simulink model "mpc_test"  (R2021b)
settings: Solver=VariableStepAuto  StartTime=0.0  StopTime=14  RelTol=1e-3
undefined symbols (not defined in the file or in its folder): carb1, carb2, carb3, carb4, carb5, DIM, KLa1, KLa2, KLa3, KLa4, LAYER, MODELTYPE, PAR1, PAR2, PAR3, PAR4, PAR5, Qin0, SETTLERINIT, SETTLERPAR, SNO2ref, SO5ref, SOSAT1, SOSAT2, SOSAT3, SOSAT4, SOSAT5, SparrowMPC_Control, T, VOL1, VOL2, VOL3, VOL4, VOL5, XINIT1, XINIT2, XINIT3, XINIT4, XINIT5, XINITDELAY
settings Model: SimulationMode=accelerator  Creator=匡  LastModifiedBy=匡
settings SolverCC: AlgebraicLoopSolver=TrustRegion
settings DataIOCC: ReturnWorkspaceOutputs=off  OutputOption=SpecifiedOutputTimes  OutputTimes=[0:1/96:14]
settings OptimizationCC: EfficientMapNaN2IntZero=off
settings DebuggingCC: InheritedTsInSrcMsg=none  UnknownTsInhSupMsg=none  SFMachineParentedDataDiag=warning  ArithmeticOperatorsInVariantConditions=warning
settings HardwareCC: TargetBitPerPointer=64  TargetBitPerSizeT=64  TargetBitPerPtrDiffT=64  TargetLongLongMode=on  TargetIntDivRoundTo=Zero  TargetEndianess=LittleEndian  TargetWordSize=64  TargetHWDeviceType=MATLAB Host  ProdEqTarget=off
settings SFSimCC: SimUseLocalCustomCode=off  CustomCodeUndefinedFunction=UseInterfaceOnly
settings RTWCC: RTWUseLocalCustomCode=off
settings CodeAppCC: MaxIdLength=128
settings GRTTargetCC: TargetLangStandard=C89/C90 (ANSI)  CombineOutputUpdateFcns=off  GRTInterface=on

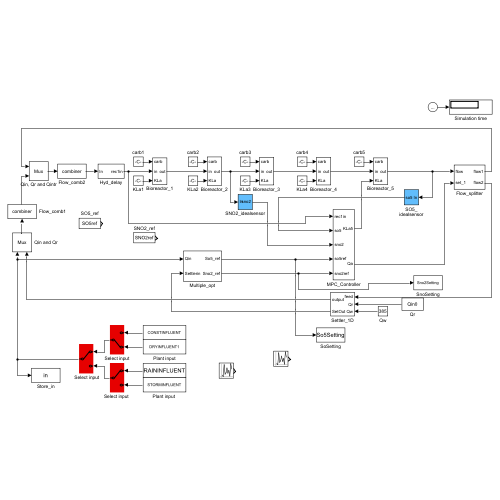
[thumbnail: Simulink's stored preview of the top-level diagram]
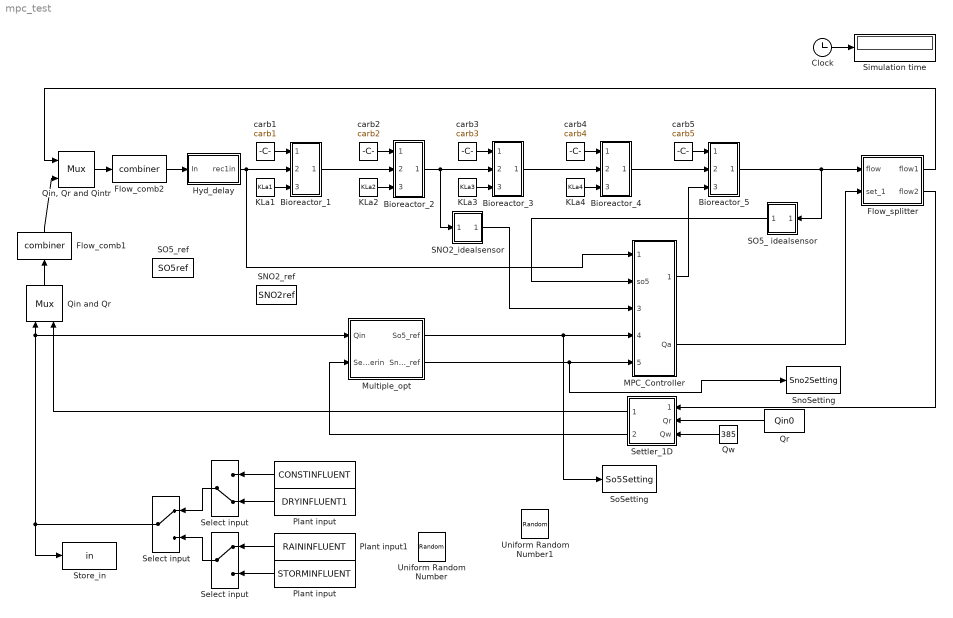
== system mpc_test ==
  " " : FromWorkspace  VariableName=CONSTINFLUENT  OutDataTypeStr=double  SampleTime=-1  ZeroCross=off  OutputAfterFinalValue=Holding final value
  " Select input" : ManualSwitch
  Bioreactor_1 : Subsystem
  Bioreactor_2 : Subsystem
  Bioreactor_3 : Subsystem
  Bioreactor_4 : Subsystem
  Bioreactor_5 : Subsystem
  Clock : Clock
  Flow_comb1 : S-Function  FunctionName=combiner  SFunctionDeploymentMode=off  EnableBusSupport=off
  Flow_comb2 : S-Function  FunctionName=combiner  SFunctionDeploymentMode=off  EnableBusSupport=off
  Flow_splitter : Subsystem
  Hyd_delay : Subsystem
  KLa1 : Constant  Value=KLa1
  KLa2 : Constant  Value=KLa2
  KLa3 : Constant  Value=KLa3
  KLa4 : Constant  Value=KLa4
  MPC_Controller : Subsystem
  Multiple_opt : Subsystem
  Plant input : FromWorkspace  VariableName=DRYINFLUENT1  SampleTime=-1  ZeroCross=off  OutputAfterFinalValue=Holding final value
  "Plant input " : FromWorkspace  VariableName=STORMINFLUENT  SampleTime=-1  ZeroCross=off  OutputAfterFinalValue=Holding final value
  Plant input1 : FromWorkspace  VariableName=RAININFLUENT  SampleTime=-1  ZeroCross=off  OutputAfterFinalValue=Holding final value
  Qin and Qr : Mux  Inputs=2
  "Qin, Qr and Qintr" : Mux  Inputs=2
  Qr : Constant  Value=Qin0
  Qw : Constant  Value=385
  SNO2_idealsensor : Subsystem
  SNO2_ref : Constant  Value=SNO2ref
  SO5_ idealsensor : Subsystem
  SO5_ref : Constant  Value=SO5ref
  Select input : ManualSwitch  CurrentSetting=0
  "Select input " : ManualSwitch
  Settler_1D : Subsystem
  Simulation time : Display
  SnoSetting : ToWorkspace  VariableName=Sno2Setting  SampleTime=1/96
  SoSetting : ToWorkspace  VariableName=So5Setting  SampleTime=1/96
  Store_in : ToWorkspace  VariableName=in  SampleTime=-1
  Uniform Random Number : UniformRandomNumber  Minimum=0.5  Maximum=2.5  Seed=547314  SampleTime=1/12
  Uniform Random Number1 : UniformRandomNumber  Minimum=0.4  Maximum=2  Seed=48658  SampleTime=1/12
  carb1 : Constant  Value=carb1
  carb2 : Constant  Value=carb2
  carb3 : Constant  Value=carb3
  carb4 : Constant  Value=carb4
  carb5 : Constant  Value=carb5
  wires:
  Settler_1D/1(output) -> Qin and Qr/2
  KLa3/1 -> Bioreactor_3/3(KLa)
  Flow_comb1/1 -> "Qin, Qr and Qintr"/2
  "Qin, Qr and Qintr"/1 -> Flow_comb2/1
  carb3/1 -> Bioreactor_3/1(carb)
  Bioreactor_1/1(out) -> Bioreactor_2/2(in)
  carb2/1 -> Bioreactor_2/1(carb)
  Plant input1/1 -> "Select input "/1
  KLa1/1 -> Bioreactor_1/3(KLa)
  carb4/1 -> Bioreactor_4/1(carb)
  Qw/1 -> Settler_1D/3(Qw)
  Bioreactor_5/1(out) -> Flow_splitter/1(flow), SO5_ idealsensor/1(In)
  KLa2/1 -> Bioreactor_2/3(KLa)
  Qin and Qr/1 -> Flow_comb1/1
  carb1/1 -> Bioreactor_1/1(carb)
  KLa4/1 -> Bioreactor_4/3(KLa)
  " "/1 -> Select input/1
  Flow_splitter/2(flow2) -> Settler_1D/1(feed)
  Flow_comb2/1 -> Hyd_delay/1(In)
  Clock/1 -> Simulation time/1
  Bioreactor_4/1(out) -> Bioreactor_5/2(in)
  "Plant input "/1 -> "Select input "/2
  Qr/1 -> Settler_1D/2(Qr)
  "Select input "/1 -> " Select input"/2
  Bioreactor_2/1(out) -> Bioreactor_3/2(in), SNO2_idealsensor/1(In)
  Select input/1 -> " Select input"/1
  Bioreactor_3/1(out) -> Bioreactor_4/2(in)
  Plant input/1 -> Select input/2
  carb5/1 -> Bioreactor_5/1(carb)
  MPC_Controller/1(KLa5) -> Bioreactor_5/3(KLa)
  MPC_Controller/2(Qa) -> Flow_splitter/2(set_1)
  SNO2_idealsensor/1(sno2) -> MPC_Controller/3(sno2)
  Hyd_delay/1(rec1in) -> MPC_Controller/1(rec1in), Bioreactor_1/2(in)
  SO5_ idealsensor/1(so5) -> MPC_Controller/2(so5)
  " Select input"/1 -> Store_in/1, Multiple_opt/1(Qin), Qin and Qr/1
  Flow_splitter/1(flow1) -> "Qin, Qr and Qintr"/1
  Settler_1D/2(SetOut) -> Multiple_opt/2(Settlerin)
  Multiple_opt/1(So5_ref) -> SoSetting/1, MPC_Controller/4(so5ref)
  Multiple_opt/2(Sno2_ref) -> SnoSetting/1, MPC_Controller/5(sno2ref)

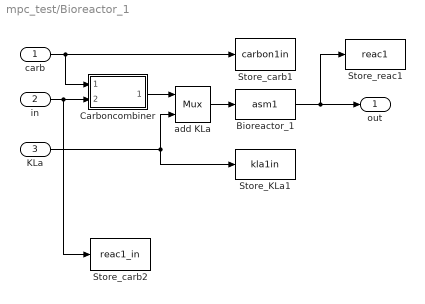
== system mpc_test/Bioreactor_1 ==
  carb : Inport
  in : Inport  Port=2
  KLa : Inport  Port=3
  Bioreactor_1 : S-Function  FunctionName=asm1  Parameters=XINIT1,PAR1,VOL1,SOSAT1  SFunctionDeploymentMode=off  EnableBusSupport=off
  Carboncombiner : Subsystem
  Store_KLa1 : ToWorkspace  VariableName=kla1in  SampleTime=-1
  Store_carb1 : ToWorkspace  VariableName=carbon1in  SampleTime=-1
  Store_carb2 : ToWorkspace  VariableName=reac1_in  SampleTime=-1
  Store_reac1 : ToWorkspace  VariableName=reac1  SampleTime=-1
  add KLa : Mux  Inputs=2
  out : Outport  VectorParamsAs1DForOutWhenUnconnected=off
  wires:
  add KLa/1 -> Bioreactor_1/1
  Bioreactor_1/1 -> out/1, Store_reac1/1
  Carboncombiner/1(Output) -> add KLa/1
  carb/1 -> Store_carb1/1, Carboncombiner/1(C_flow)
  in/1 -> Store_carb2/1, Carboncombiner/2(Input)
  KLa/1 -> add KLa/2, Store_KLa1/1

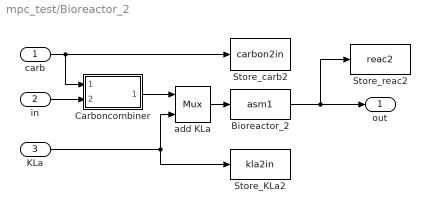
== system mpc_test/Bioreactor_2 ==
  carb : Inport
  in : Inport  Port=2
  KLa : Inport  Port=3
  Bioreactor_2 : S-Function  FunctionName=asm1  Parameters=XINIT2,PAR2,VOL2,SOSAT2  SFunctionDeploymentMode=off  EnableBusSupport=off
  Carboncombiner : Subsystem
  Store_KLa2 : ToWorkspace  VariableName=kla2in  SampleTime=-1
  Store_carb2 : ToWorkspace  VariableName=carbon2in  SampleTime=-1
  Store_reac2 : ToWorkspace  VariableName=reac2  SampleTime=-1
  add KLa : Mux  Inputs=2
  out : Outport  VectorParamsAs1DForOutWhenUnconnected=off
  wires:
  Bioreactor_2/1 -> out/1, Store_reac2/1
  add KLa/1 -> Bioreactor_2/1
  Carboncombiner/1(Output) -> add KLa/1
  carb/1 -> Carboncombiner/1(C_flow), Store_carb2/1
  in/1 -> Carboncombiner/2(Input)
  KLa/1 -> add KLa/2, Store_KLa2/1

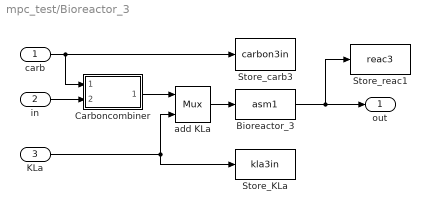
== system mpc_test/Bioreactor_3 ==
  carb : Inport
  in : Inport  Port=2
  KLa : Inport  Port=3
  Bioreactor_3 : S-Function  FunctionName=asm1  Parameters=XINIT3,PAR3,VOL3,SOSAT3  SFunctionDeploymentMode=off  EnableBusSupport=off
  Carboncombiner : Subsystem
  Store_KLa : ToWorkspace  VariableName=kla3in  SampleTime=-1
  Store_carb3 : ToWorkspace  VariableName=carbon3in  SampleTime=-1
  Store_reac1 : ToWorkspace  VariableName=reac3  SampleTime=-1
  add KLa : Mux  Inputs=2
  out : Outport  VectorParamsAs1DForOutWhenUnconnected=off
  wires:
  Bioreactor_3/1 -> out/1, Store_reac1/1
  add KLa/1 -> Bioreactor_3/1
  Carboncombiner/1(Output) -> add KLa/1
  carb/1 -> Carboncombiner/1(C_flow), Store_carb3/1
  in/1 -> Carboncombiner/2(Input)
  KLa/1 -> add KLa/2, Store_KLa/1

== system mpc_test/Bioreactor_4 ==
  carb : Inport
  in : Inport  Port=2
  KLa : Inport  Port=3
  Bioreactor_4 : S-Function  FunctionName=asm1  Parameters=XINIT4,PAR4,VOL4,SOSAT4  SFunctionDeploymentMode=off  EnableBusSupport=off
  Carboncombiner : Subsystem
  Store_KLa4 : ToWorkspace  VariableName=kla4in  SampleTime=-1
  Store_carb4 : ToWorkspace  VariableName=carbon4in  SampleTime=-1
  Store_reac4 : ToWorkspace  VariableName=reac4  SampleTime=-1
  add KLa : Mux  Inputs=2
  out : Outport  VectorParamsAs1DForOutWhenUnconnected=off
  wires:
  Bioreactor_4/1 -> out/1, Store_reac4/1
  add KLa/1 -> Bioreactor_4/1
  Carboncombiner/1(Output) -> add KLa/1
  carb/1 -> Carboncombiner/1(C_flow), Store_carb4/1
  in/1 -> Carboncombiner/2(Input)
  KLa/1 -> add KLa/2, Store_KLa4/1

== system mpc_test/Bioreactor_5 ==
  carb : Inport
  in : Inport  Port=2
  KLa : Inport  Port=3
  Bioreactor_5 : S-Function  FunctionName=asm1  Parameters=XINIT5,PAR5,VOL5,SOSAT5  SFunctionDeploymentMode=off  EnableBusSupport=off
  Carboncombiner : Subsystem
  Store_KLa5 : ToWorkspace  VariableName=kla5in  SampleTime=-1
  Store_carb5 : ToWorkspace  VariableName=carbon5in  SampleTime=-1
  Store_reac5 : ToWorkspace  VariableName=reac5  SampleTime=-1
  add KLa : Mux  Inputs=2
  out : Outport  VectorParamsAs1DForOutWhenUnconnected=off
  wires:
  Bioreactor_5/1 -> out/1, Store_reac5/1
  add KLa/1 -> Bioreactor_5/1
  Carboncombiner/1(Output) -> add KLa/1
  carb/1 -> Carboncombiner/1(C_flow), Store_carb5/1
  in/1 -> Carboncombiner/2(Input)
  KLa/1 -> Store_KLa5/1, add KLa/2

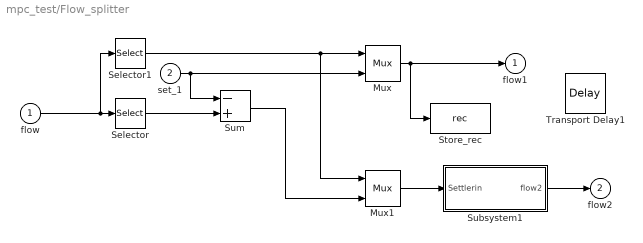
== system mpc_test/Flow_splitter ==
  flow : Inport
  set_1 : Inport  Port=2
  Mux : Mux  Inputs=2
  Mux1 : Mux  Inputs=2
  Selector : Selector  InputPortWidth=15  IndexOptions=Index vector (dialog)  Indices=[15]  OutputSizes=1
  Selector1 : Selector  InputPortWidth=15  IndexOptions=Index vector (dialog)  Indices=[1 2 3 4 5 6 7 8 9 10 11 12 13 14]  OutputSizes=1
  Store_rec : ToWorkspace  VariableName=rec  SampleTime=-1
  Subsystem1 : Subsystem
  Sum : Sum  Inputs=-+  InputSameDT=on  SaturateOnIntegerOverflow=on  OutDataTypeStr=Inherit: Same as first input
  Transport Delay1 : TransportDelay  DelayTime=0.000002  InitialOutput=18460
  flow1 : Outport  VectorParamsAs1DForOutWhenUnconnected=off
  flow2 : Outport  Port=2  VectorParamsAs1DForOutWhenUnconnected=off
  wires:
  flow/1 -> Selector1/1, Selector/1
  set_1/1 -> Mux/2, Sum/1
  Selector/1 -> Sum/2
  Sum/1 -> Mux1/2
  Selector1/1 -> Mux/1, Mux1/1
  Mux/1 -> flow1/1, Store_rec/1
  Mux1/1 -> Subsystem1/1(Settlerin)
  Subsystem1/1(flow2) -> flow2/1

== system mpc_test/Hyd_delay ==
  In : Inport
  Demux : Demux  Outputs=[14,1]
      settings: DisplayOption=none
  Hyd_delay : S-Function  FunctionName=hyddelayv3  Parameters=XINITDELAY,PAR1,T  SFunctionDeploymentMode=off  EnableBusSupport=off
  Mux : Mux  Inputs=2
  Product : Product  SaturateOnIntegerOverflow=on  OutDataTypeStr=Inherit: Same as first input
  Store_ASinput : ToWorkspace  VariableName=ASinput  SampleTime=-1
  rec1in : Outport  VectorParamsAs1DForOutWhenUnconnected=off
  wires:
  In/1 -> Hyd_delay/1
  Hyd_delay/1 -> rec1in/1, Demux/1
  Demux/1 -> Product/1
  Demux/2 -> Product/2, Mux/2
  Product/1 -> Mux/1
  Mux/1 -> Store_ASinput/1

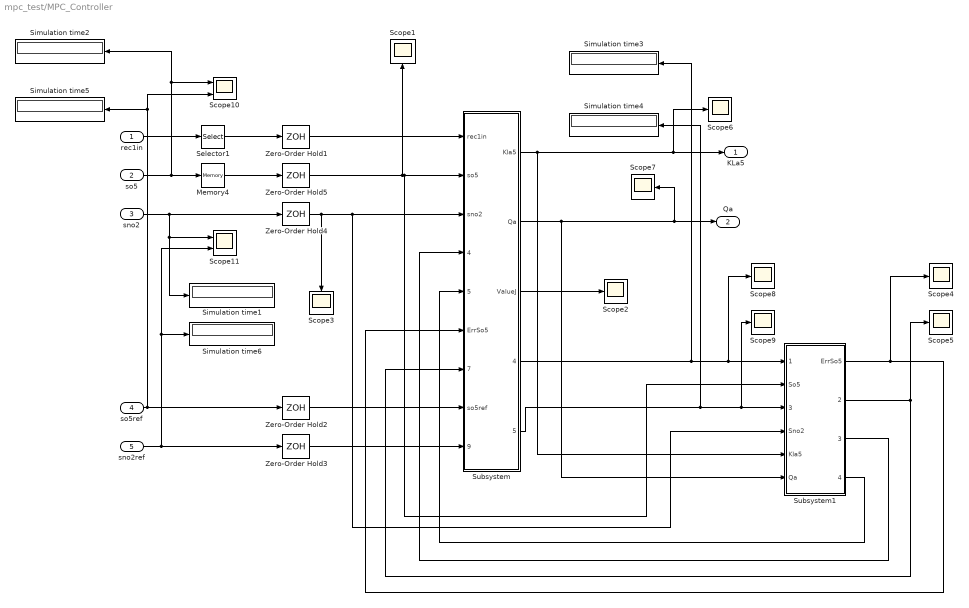
== system mpc_test/MPC_Controller ==
  rec1in : Inport
  so5 : Inport  Port=2
  sno2 : Inport  Port=3
  so5ref : Inport  Port=4
  sno2ref : Inport  Port=5
  Memory4 : Memory  InitialCondition=2  InheritSampleTime=on
  Scope{1..9} (9 alike) : Scope
  Scope10 : Scope  NumInputPorts=2
  Scope11 : Scope  NumInputPorts=2
  Selector1 : Selector  InputPortWidth=15  IndexOptions=Index vector (dialog)  Indices=[1:15]  OutputSizes=1
  Simulation time{1..6} (6 alike) : Display
  Subsystem : Subsystem
  Subsystem1 : Subsystem
  Zero-Order Hold{1..5} (5 alike) : ZeroOrderHold  SampleTime=1/288
  KLa5 : Outport  VectorParamsAs1DForOutWhenUnconnected=off
  Qa : Outport  Port=2  VectorParamsAs1DForOutWhenUnconnected=off
  wires:
  so5/1 -> Simulation time2/1, Scope10/1, Memory4/1
  so5ref/1 -> Scope10/2, Simulation time5/1, Zero-Order Hold2/1
  Subsystem/2(Qa) -> Subsystem1/6(Qa), Qa/1, Scope7/1
  Subsystem/3(ValueJ) -> Scope2/1
  Subsystem1/1(ErrSo5) -> Scope4/1, Subsystem/6(ErrSo5)
  Subsystem1/2(ErrSno2) -> Subsystem/7(ErrSno2), Scope5/1
  Zero-Order Hold2/1 -> Subsystem/8(so5ref)
  Zero-Order Hold3/1 -> Subsystem/9(sno2ref)
  rec1in/1 -> Selector1/1
  Memory4/1 -> Zero-Order Hold5/1
  Zero-Order Hold1/1 -> Subsystem/1(rec1in)
  Zero-Order Hold5/1 -> Subsystem/2(so5), Subsystem1/2(So5), Scope1/1
  sno2/1 -> Zero-Order Hold4/1, Simulation time1/1, Scope11/1
  Subsystem1/3(DelayKla5) -> Subsystem/4(DelayKla5)
  Subsystem1/4(DelayQa) -> Subsystem/5(DelayQa)
  Selector1/1 -> Zero-Order Hold1/1
  Subsystem/4(PredSo5) -> Scope8/1, Subsystem1/1(PredSo5), Simulation time3/1
  Subsystem/5(PredSno2) -> Scope9/1, Subsystem1/3(PredSno2), Simulation time4/1
  Subsystem/1(Kla5) -> Scope6/1, KLa5/1, Subsystem1/5(Kla5)
  Zero-Order Hold4/1 -> Scope3/1, Subsystem1/4(Sno2), Subsystem/3(sno2)
  sno2ref/1 -> Scope11/2, Simulation time6/1, Zero-Order Hold3/1

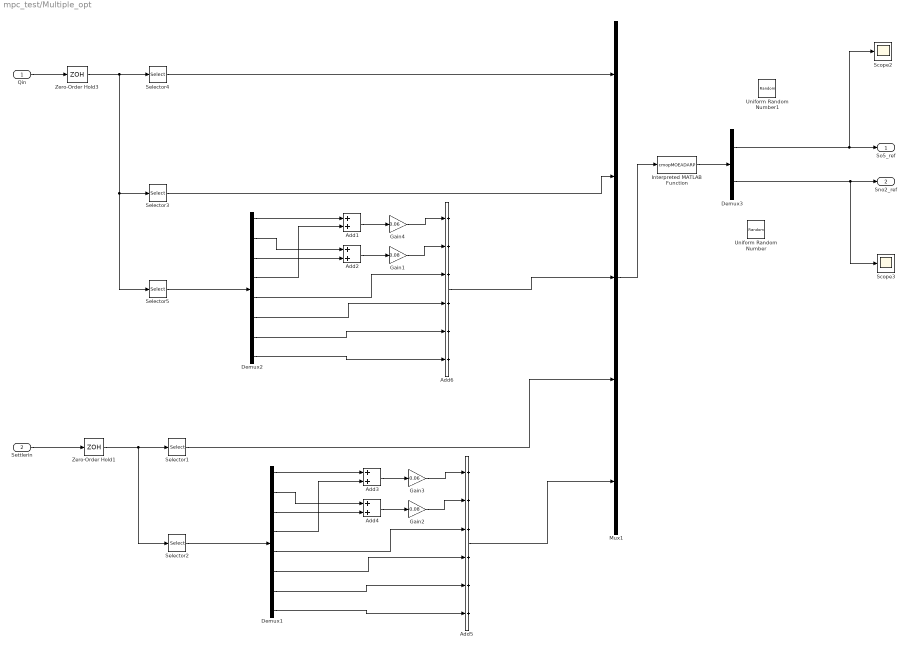
== system mpc_test/Multiple_opt ==
  Qin : Inport
  Settlerin : Inport  Port=2
  Add{1..4} (4 alike) : Sum
  Add5 : Sum  Inputs=++++++
  Add6 : Sum  Inputs=++++++
  Demux1 : Demux  Outputs=8
  Demux2 : Demux  Outputs=8
  Demux3 : Demux  Outputs=2
  Gain1 : Gain  Gain=0.08
  Gain2 : Gain  Gain=0.08
  Gain3 : Gain  Gain=0.06
  Gain4 : Gain  Gain=0.06
  Interpreted MATLAB Function : MATLABFcn  MATLABFcn=cmopMOEADARP  OutputDimensions=2
  Mux1 : Mux  Inputs=5
  Scope2 : Scope
  Scope3 : Scope
  Selector1 : Selector  InputPortWidth=15  IndexOptions=Index vector (dialog)  Indices=[10]  OutputSizes=1
  Selector2 : Selector  InputPortWidth=15  IndexOptions=Index vector (dialog)  Indices=[3 ,5:7,9:12]  OutputSizes=1
  Selector3 : Selector  InputPortWidth=15  IndexOptions=Index vector (dialog)  Indices=[10]  OutputSizes=1
  Selector4 : Selector  InputPortWidth=15  IndexOptions=Index vector (dialog)  Indices=[15]  OutputSizes=1
  Selector5 : Selector  InputPortWidth=15  IndexOptions=Index vector (dialog)  Indices=[3 ,5:7,9:12]  OutputSizes=1
  Uniform Random Number : UniformRandomNumber  Minimum=-0.5  Maximum=0.5  Seed=5645465  SampleTime=1
  Uniform Random Number1 : UniformRandomNumber  Seed=487842361  SampleTime=1
  Zero-Order Hold1 : ZeroOrderHold  SampleTime=1/12
  Zero-Order Hold3 : ZeroOrderHold  SampleTime=1/12
  So5_ref : Outport  VectorParamsAs1DForOutWhenUnconnected=off
  Sno2_ref : Outport  Port=2  VectorParamsAs1DForOutWhenUnconnected=off
  wires:
  Mux1/1 -> Interpreted MATLAB Function/1
  Interpreted MATLAB Function/1 -> Demux3/1
  Qin/1 -> Zero-Order Hold3/1
  Demux1/7 -> Add5/5
  Demux1/1 -> Add3/1
  Demux1/4 -> Add3/2
  Demux1/3 -> Add4/2
  Demux1/2 -> Add4/1
  Gain3/1 -> Add5/1
  Demux1/6 -> Add5/4
  Demux1/5 -> Add5/3
  Demux1/8 -> Add5/6
  Gain2/1 -> Add5/2
  Add3/1 -> Gain3/1
  Selector2/1 -> Demux1/1
  Add4/1 -> Gain2/1
  Zero-Order Hold1/1 -> Selector2/1, Selector1/1
  Settlerin/1 -> Zero-Order Hold1/1
  Selector1/1 -> Mux1/4
  Add5/1 -> Mux1/5
  Selector4/1 -> Mux1/1
  Gain1/1 -> Add6/2
  Demux2/6 -> Add6/4
  Demux2/2 -> Add2/1
  Selector5/1 -> Demux2/1
  Selector3/1 -> Mux1/2
  Demux2/7 -> Add6/5
  Add1/1 -> Gain4/1
  Gain4/1 -> Add6/1
  Add6/1 -> Mux1/3
  Add2/1 -> Gain1/1
  Demux2/8 -> Add6/6
  Zero-Order Hold3/1 -> Selector5/1, Selector3/1, Selector4/1
  Demux2/1 -> Add1/1
  Demux2/5 -> Add6/3
  Demux2/4 -> Add1/2
  Demux2/3 -> Add2/2
  Demux3/1 -> Scope2/1, So5_ref/1
  Demux3/2 -> Scope3/1, Sno2_ref/1

== system mpc_test/SNO2_idealsensor ==
  In : Inport
  Mux : Mux  Inputs=6
  Selector : Selector  InputPortWidth=15  IndexOptions=Index vector (dialog)  Indices=[9]  OutputSizes=1
  To Workspace : ToWorkspace  VariableName=SNO2sensor  SampleTime=-1
  sno2 : Outport  VectorParamsAs1DForOutWhenUnconnected=off
  wires:
  Selector/1 -> Mux/3, Mux/4, sno2/1, Mux/5, Mux/6, Mux/2, Mux/1
  In/1 -> Selector/1
  Mux/1 -> To Workspace/1

== system mpc_test/SO5_ idealsensor ==
  In : Inport
  Mux : Mux  Inputs=6
  Selector : Selector  InputPortWidth=15  IndexOptions=Index vector (dialog)  Indices=[8]  OutputSizes=1
  To Workspace : ToWorkspace  VariableName=SO5sensor  SampleTime=-1
  so5 : Outport  VectorParamsAs1DForOutWhenUnconnected=off
  wires:
  Selector/1 -> Mux/3, Mux/4, so5/1, Mux/5, Mux/6, Mux/2, Mux/1
  In/1 -> Selector/1
  Mux/1 -> To Workspace/1

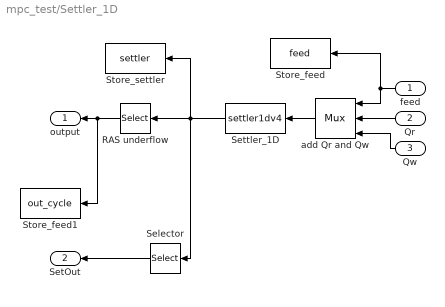
== system mpc_test/Settler_1D ==
  feed : Inport
  Qr : Inport  Port=2
  Qw : Inport  Port=3
  RAS underflow : Selector  InputPortWidth=113  IndexOptions=Index vector (dialog)  Indices=[1 2 3 4 5 6 7 8 9 10 11 12 13 14 15]  OutputSizes=1
  Selector : Selector  InputPortWidth=113  IndexOptions=Index vector (dialog)  Indices=[17:31]  OutputSizes=1
  Settler_1D : S-Function  FunctionName=settler1dv4  Parameters=SETTLERINIT,SETTLERPAR,DIM,LAYER,MODELTYPE  SFunctionDeploymentMode=off  EnableBusSupport=off
  Store_feed : ToWorkspace  VariableName=feed  SampleTime=-1
  Store_feed1 : ToWorkspace  VariableName=out_cycle  SampleTime=-1
  Store_settler : ToWorkspace  VariableName=settler  SampleTime=-1
  add Qr and Qw : Mux  Inputs=3
  output : Outport  VectorParamsAs1DForOutWhenUnconnected=off
  SetOut : Outport  Port=2  VectorParamsAs1DForOutWhenUnconnected=off
  wires:
  add Qr and Qw/1 -> Settler_1D/1
  Qr/1 -> add Qr and Qw/2
  Qw/1 -> add Qr and Qw/3
  feed/1 -> add Qr and Qw/1, Store_feed/1
  RAS underflow/1 -> Store_feed1/1, output/1
  Settler_1D/1 -> Selector/1, RAS underflow/1, Store_settler/1
  Selector/1 -> SetOut/1

== system mpc_test/Bioreactor_1/Carboncombiner ==
  C_flow : Inport
  Input : Inport  Port=2
  Carboncombiner : S-Function  FunctionName=carboncombiner  Parameters=CARBONSOURCECONC  SFunctionDeploymentMode=off  EnableBusSupport=off
  Mux : Mux  Inputs=2
  Output : Outport  VectorParamsAs1DForOutWhenUnconnected=off
  wires:
  C_flow/1 -> Mux/1
  Mux/1 -> Carboncombiner/1
  Carboncombiner/1 -> Output/1
  Input/1 -> Mux/2

== system mpc_test/Bioreactor_2/Carboncombiner ==
  C_flow : Inport
  Input : Inport  Port=2
  Carboncombiner : S-Function  FunctionName=carboncombiner  Parameters=CARBONSOURCECONC  SFunctionDeploymentMode=off  EnableBusSupport=off
  Mux : Mux  Inputs=2
  Output : Outport  VectorParamsAs1DForOutWhenUnconnected=off
  wires:
  Input/1 -> Mux/2
  Carboncombiner/1 -> Output/1
  Mux/1 -> Carboncombiner/1
  C_flow/1 -> Mux/1

== system mpc_test/Bioreactor_3/Carboncombiner ==
  C_flow : Inport
  Input : Inport  Port=2
  Carboncombiner : S-Function  FunctionName=carboncombiner  Parameters=CARBONSOURCECONC  SFunctionDeploymentMode=off  EnableBusSupport=off
  Mux : Mux  Inputs=2
  Output : Outport  VectorParamsAs1DForOutWhenUnconnected=off
  wires:
  Input/1 -> Mux/2
  Carboncombiner/1 -> Output/1
  Mux/1 -> Carboncombiner/1
  C_flow/1 -> Mux/1

== system mpc_test/Bioreactor_4/Carboncombiner ==
  C_flow : Inport
  Input : Inport  Port=2
  Carboncombiner : S-Function  FunctionName=carboncombiner  Parameters=CARBONSOURCECONC  SFunctionDeploymentMode=off  EnableBusSupport=off
  Mux : Mux  Inputs=2
  Output : Outport  VectorParamsAs1DForOutWhenUnconnected=off
  wires:
  Input/1 -> Mux/2
  Carboncombiner/1 -> Output/1
  Mux/1 -> Carboncombiner/1
  C_flow/1 -> Mux/1

== system mpc_test/Bioreactor_5/Carboncombiner ==
  C_flow : Inport
  Input : Inport  Port=2
  Carboncombiner : S-Function  FunctionName=carboncombiner  Parameters=CARBONSOURCECONC  SFunctionDeploymentMode=off  EnableBusSupport=off
  Mux : Mux  Inputs=2
  Output : Outport  VectorParamsAs1DForOutWhenUnconnected=off
  wires:
  Input/1 -> Mux/2
  Carboncombiner/1 -> Output/1
  Mux/1 -> Carboncombiner/1
  C_flow/1 -> Mux/1

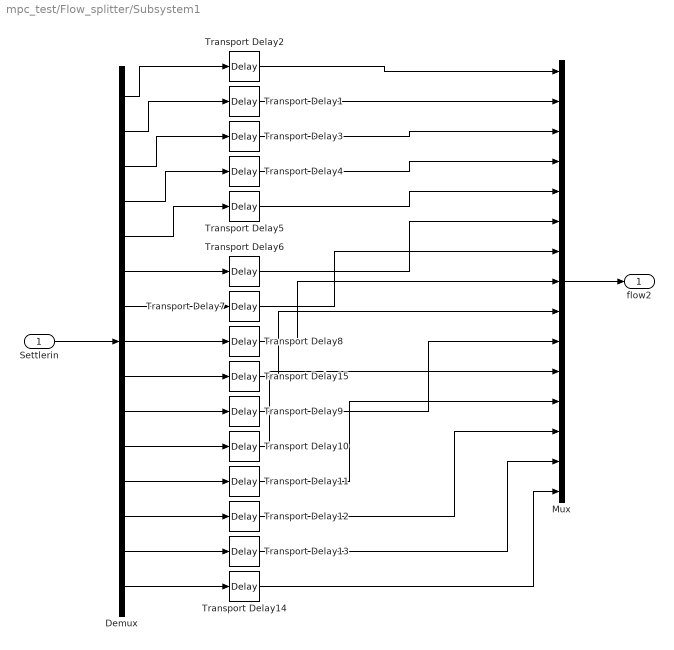
== system mpc_test/Flow_splitter/Subsystem1 ==
  Settlerin : Inport
  Demux : Demux  Outputs=15
  Mux : Mux  Inputs=15
  Transport Delay1 : TransportDelay  DelayTime=0.000002  InitialOutput=0.8895
  Transport Delay10 : TransportDelay  DelayTime=0.000002  InitialOutput=0.6883
  Transport Delay11 : TransportDelay  DelayTime=0.000002  InitialOutput=0.0135
  Transport Delay12 : TransportDelay  DelayTime=0.000002  InitialOutput=4.1256
  Transport Delay13 : TransportDelay  DelayTime=0.000002  InitialOutput=12.4969
  Transport Delay14 : TransportDelay  DelayTime=0.000002  InitialOutput=73393
  Transport Delay15 : TransportDelay  DelayTime=0.000002  InitialOutput=10.4125
  Transport Delay2 : TransportDelay  DelayTime=0.000002  InitialOutput=30
  Transport Delay3 : TransportDelay  DelayTime=0.000002  InitialOutput=4.3918
  Transport Delay4 : TransportDelay  DelayTime=0.000002  InitialOutput=0.1884
  Transport Delay5 : TransportDelay  DelayTime=0.000002  InitialOutput=9.7815
  Transport Delay6 : TransportDelay  DelayTime=0.000002  InitialOutput=0.5725
  Transport Delay7 : TransportDelay  DelayTime=0.000002  InitialOutput=1.7283
  Transport Delay8 : TransportDelay  DelayTime=0.000002  InitialOutput=0.4909
  Transport Delay9 : TransportDelay  DelayTime=0.000002  InitialOutput=1.7333
  flow2 : Outport
  wires:
  Demux/1 -> Transport Delay2/1
  Demux/2 -> Transport Delay1/1
  Demux/3 -> Transport Delay3/1
  Demux/4 -> Transport Delay4/1
  Demux/5 -> Transport Delay5/1
  Demux/6 -> Transport Delay6/1
  Demux/7 -> Transport Delay7/1
  Settlerin/1 -> Demux/1
  Transport Delay2/1 -> Mux/1
  Transport Delay1/1 -> Mux/2
  Transport Delay3/1 -> Mux/3
  Transport Delay4/1 -> Mux/4
  Transport Delay5/1 -> Mux/5
  Mux/1 -> flow2/1
  Demux/15 -> Transport Delay14/1
  Demux/14 -> Transport Delay13/1
  Demux/13 -> Transport Delay12/1
  Demux/12 -> Transport Delay11/1
  Demux/11 -> Transport Delay10/1
  Demux/10 -> Transport Delay9/1
  Demux/9 -> Transport Delay15/1
  Demux/8 -> Transport Delay8/1
  Transport Delay6/1 -> Mux/6
  Transport Delay7/1 -> Mux/7
  Transport Delay8/1 -> Mux/8
  Transport Delay15/1 -> Mux/9
  Transport Delay9/1 -> Mux/10
  Transport Delay10/1 -> Mux/11
  Transport Delay11/1 -> Mux/12
  Transport Delay12/1 -> Mux/13
  Transport Delay13/1 -> Mux/14
  Transport Delay14/1 -> Mux/15

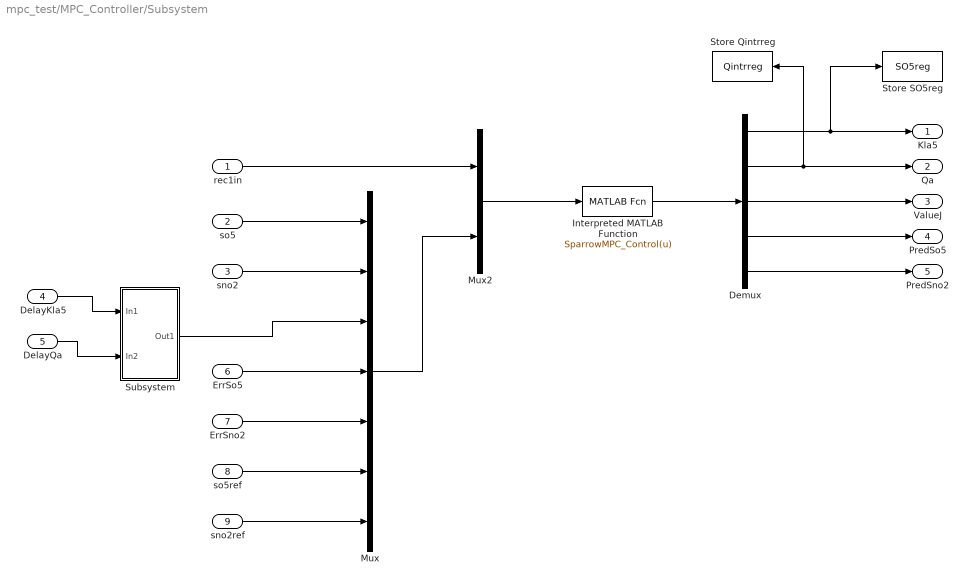
== system mpc_test/MPC_Controller/Subsystem ==
  rec1in : Inport
  so5 : Inport  Port=2
  sno2 : Inport  Port=3
  DelayKla5 : Inport  Port=4
  DelayQa : Inport  Port=5
  ErrSo5 : Inport  Port=6
  ErrSno2 : Inport  Port=7
  so5ref : Inport  Port=8
  sno2ref : Inport  Port=9
  Demux : Demux  Outputs=5
  Interpreted MATLAB Function : MATLABFcn  MATLABFcn=SparrowMPC_Control(u)  OutputDimensions=5
  Mux : Mux  Inputs=7
  Mux2 : Mux  Inputs=2
  Store Qintrreg : ToWorkspace  VariableName=Qintrreg  SampleTime=-1
  Store SO5reg : ToWorkspace  VariableName=SO5reg  SampleTime=-1
  Subsystem : Subsystem
  Kla5 : Outport  VectorParamsAs1DForOutWhenUnconnected=off
  Qa : Outport  Port=2  VectorParamsAs1DForOutWhenUnconnected=off
  ValueJ : Outport  Port=3  VectorParamsAs1DForOutWhenUnconnected=off
  PredSo5 : Outport  Port=4  VectorParamsAs1DForOutWhenUnconnected=off
  PredSno2 : Outport  Port=5  VectorParamsAs1DForOutWhenUnconnected=off
  wires:
  Mux2/1 -> Interpreted MATLAB Function/1
  Mux/1 -> Mux2/2
  rec1in/1 -> Mux2/1
  so5/1 -> Mux/1
  sno2/1 -> Mux/2
  Subsystem/1(Out1) -> Mux/3
  ErrSo5/1 -> Mux/4
  ErrSno2/1 -> Mux/5
  so5ref/1 -> Mux/6
  Interpreted MATLAB Function/1 -> Demux/1
  Demux/1 -> Store SO5reg/1, Kla5/1
  Demux/2 -> Store Qintrreg/1, Qa/1
  Demux/3 -> ValueJ/1
  Demux/4 -> PredSo5/1
  Demux/5 -> PredSno2/1
  DelayKla5/1 -> Subsystem/1(In1)
  DelayQa/1 -> Subsystem/2(In2)
  sno2ref/1 -> Mux/7

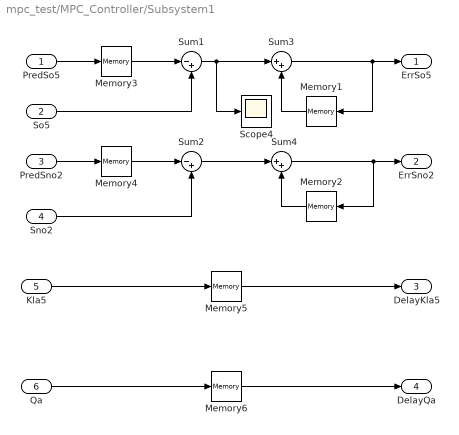
== system mpc_test/MPC_Controller/Subsystem1 ==
  PredSo5 : Inport
  So5 : Inport  Port=2
  PredSno2 : Inport  Port=3
  Sno2 : Inport  Port=4
  Kla5 : Inport  Port=5
  Qa : Inport  Port=6
  Memory1 : Memory  InheritSampleTime=on
  Memory2 : Memory  InheritSampleTime=on
  Memory3 : Memory  InitialCondition=2  InheritSampleTime=on
  Memory4 : Memory  InitialCondition=1  InheritSampleTime=on
  Memory5 : Memory  InitialCondition=84  InheritSampleTime=on
  Memory6 : Memory  InitialCondition=55338  InheritSampleTime=on
  Scope4 : Scope
  Sum1 : Sum  Inputs=|-+
  Sum2 : Sum  Inputs=|-+
  Sum3 : Sum  Inputs=|++
  Sum4 : Sum  Inputs=|++
  ErrSo5 : Outport  VectorParamsAs1DForOutWhenUnconnected=off
  ErrSno2 : Outport  Port=2  VectorParamsAs1DForOutWhenUnconnected=off
  DelayKla5 : Outport  Port=3  VectorParamsAs1DForOutWhenUnconnected=off
  DelayQa : Outport  Port=4  VectorParamsAs1DForOutWhenUnconnected=off
  wires:
  PredSo5/1 -> Memory3/1
  PredSno2/1 -> Memory4/1
  Memory5/1 -> DelayKla5/1
  Memory6/1 -> DelayQa/1
  Kla5/1 -> Memory5/1
  Qa/1 -> Memory6/1
  So5/1 -> Sum1/2
  Sno2/1 -> Sum2/2
  Memory3/1 -> Sum1/1
  Memory4/1 -> Sum2/1
  Sum3/1 -> ErrSo5/1, Memory1/1
  Memory1/1 -> Sum3/2
  Memory2/1 -> Sum4/2
  Sum4/1 -> ErrSno2/1, Memory2/1
  Sum1/1 -> Scope4/1, Sum3/1
  Sum2/1 -> Sum4/1

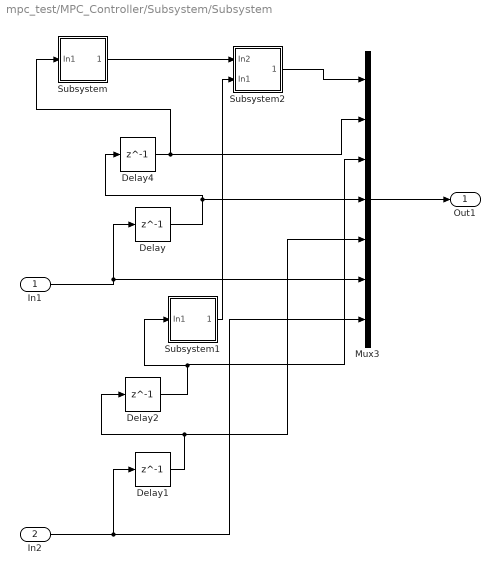
== system mpc_test/MPC_Controller/Subsystem/Subsystem ==
  In1 : Inport
  In2 : Inport  Port=2
  Delay : Delay  DelayLength=1  InitialCondition=84
  Delay1 : Delay  DelayLength=1  InitialCondition=55338
  Delay2 : Delay  DelayLength=1  InitialCondition=55338
  Delay4 : Delay  DelayLength=1  InitialCondition=84
  Mux3 : Mux  Inputs=7
  Subsystem : Subsystem
  Subsystem1 : Subsystem
  Subsystem2 : Subsystem
  Out1 : Outport  VectorParamsAs1DForOutWhenUnconnected=off
  wires:
  In2/1 -> Mux3/7, Delay1/1
  Delay2/1 -> Subsystem1/1(In1), Mux3/3
  In1/1 -> Delay/1, Mux3/6
  Delay/1 -> Delay4/1, Mux3/4
  Delay4/1 -> Subsystem/1(In1), Mux3/2
  Mux3/1 -> Out1/1
  Delay1/1 -> Mux3/5, Delay2/1
  Subsystem1/1(Out1) -> Subsystem2/2(In1)
  Subsystem/1(Out1) -> Subsystem2/1(In2)
  Subsystem2/1(Out1) -> Mux3/1

== system mpc_test/MPC_Controller/Subsystem/Subsystem/Subsystem ==
  In1 : Inport
  Delay : Delay  DelayLength=1  InitialCondition=84
  Out1 : Outport
  wires:
  In1/1 -> Delay/1
  Delay/1 -> Out1/1

== system mpc_test/MPC_Controller/Subsystem/Subsystem/Subsystem1 ==
  In1 : Inport
  Delay : Delay  DelayLength=1  InitialCondition=55338
  Out1 : Outport
  wires:
  In1/1 -> Delay/1
  Delay/1 -> Out1/1

== system mpc_test/MPC_Controller/Subsystem/Subsystem/Subsystem2 ==
  In2 : Inport
  In1 : Inport  Port=2
  Mux : Mux  Inputs=2
  Out1 : Outport
  wires:
  Mux/1 -> Out1/1
  In1/1 -> Mux/2
  In2/1 -> Mux/1
